simulink model "safety"  (R2014a)
settings: Solver=FixedStepDiscrete  StartTime=0.0  StopTime=inf  FixedStep=2.5e-4  RelTol=1e-3
libraries: simulink x10, xpcethercatlib x5
settings Model: xpc_rtwmakecfg_data=_xpcethercatlib_  Creator=drl  LastModifiedBy=drl
settings OptimizationCC: BlockReduction=off

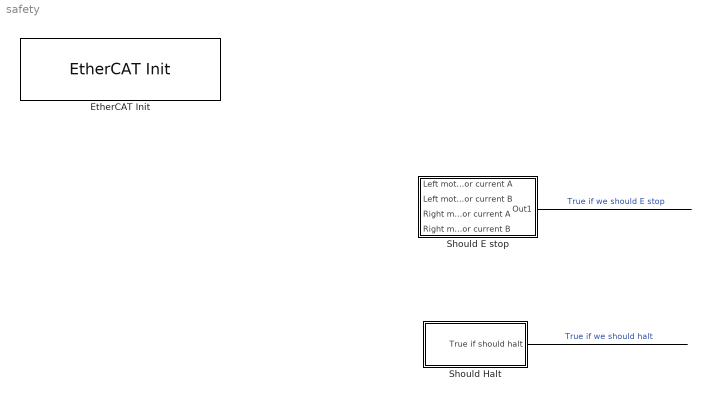
== system safety ==
  "EtherCAT Init " : xpcethercatlib/EtherCAT Init   Priority=0  config_file=C:\Users\drl\Documents\MATLAB\eni_elmo_medulla_4khz.xml  device_id=0  pci_bus=0  pci_slot=0  enaDebug=off  enaDC=on  errLink=off  masterDbg=off  stateChgDbg=off  baseClock=off  masterCfg=off  logFile='c:\dbglog.txt'  sample_time=0.000250
  Should E stop : Subsystem
  Should Halt : Subsystem
  wires:
  Should Halt/1(True if should halt) -> ?  "True if we should halt"
  Should E stop/1(Out1) -> ?  "True if we should E stop"

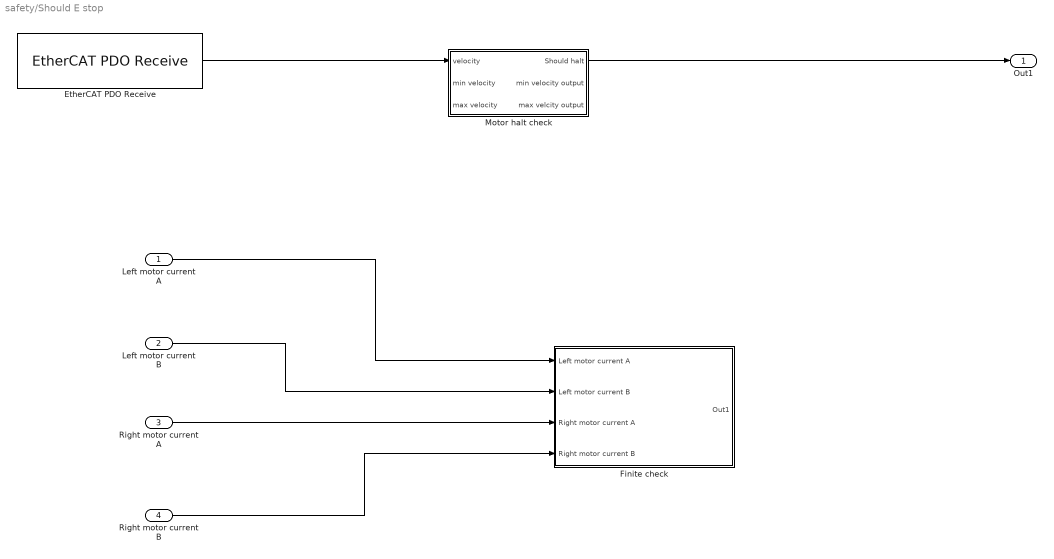
== system safety/Should E stop ==
  Left motor current A : Inport
  Left motor current B : Inport  Port=2
  Right motor current A : Inport  Port=3
  Right motor current B : Inport  Port=4
  EtherCAT PDO Receive : xpcethercatlib/EtherCAT PDO Receive  Priority=2  sig_name=Box 1 (Elmo Drive).Inputs.Position actual value  sig_offset=1064  sig_type=int32  type_size=32  sig_dim=1  device_id=0  sample_time=0.00025
  Finite check : Subsystem
  Motor halt check : Subsystem
  Out1 : Outport
  wires:
  Motor halt check/1(Should halt) -> Out1/1
  EtherCAT PDO Receive/1 -> Motor halt check/1(velocity)
  Left motor current A/1 -> Finite check/1(Left motor current A)
  Left motor current B/1 -> Finite check/2(Left motor current B)
  Right motor current A/1 -> Finite check/3(Right motor current A)
  Right motor current B/1 -> Finite check/4(Right motor current B)

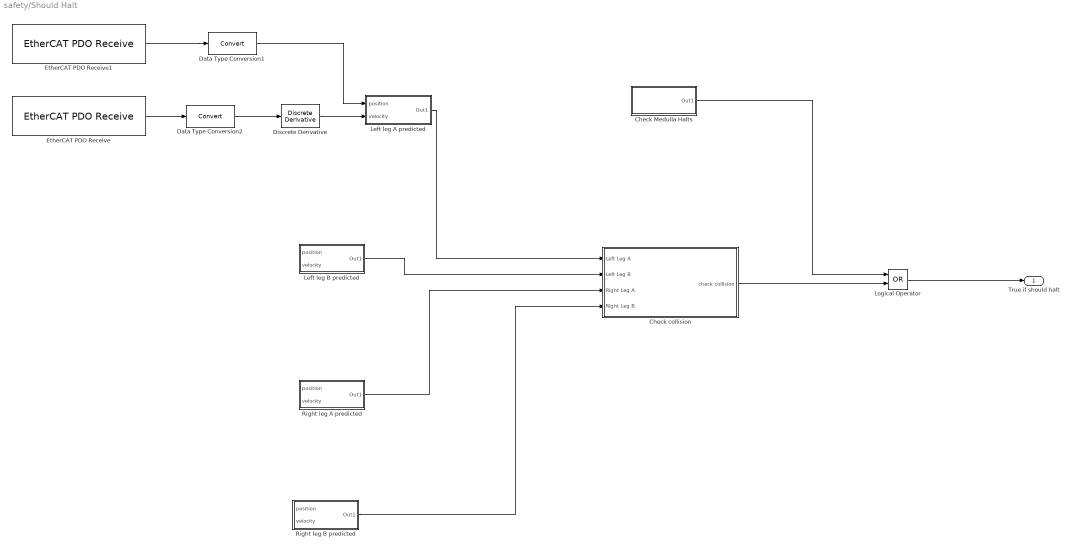
== system safety/Should Halt ==
  Check Medulla Halts : Subsystem
  Check collision : Subsystem
  Data Type Conversion1 : DataTypeConversion
  Data Type Conversion2 : DataTypeConversion
  Discrete Derivative : simulink/Discrete/Discrete Derivative  gainval=1.0  ICPrevScaledInput=0.0  InputProcessing=Inherited  OutMin=[]  OutMax=[]  OutDataType=fixdt(1, 16)  OutScaling=2^-10  DoSatur=off
  EtherCAT PDO Receive : xpcethercatlib/EtherCAT PDO Receive  Priority=2  sig_name=Box 1 (Elmo Drive).Inputs.Position actual value  sig_offset=1064  sig_type=int32  type_size=32  sig_dim=1  device_id=0  sample_time=0.00025
  EtherCAT PDO Receive1 : xpcethercatlib/EtherCAT PDO Receive  Priority=2  sig_name=Drive 1 (Elmo Drive).Inputs.Position actual value  sig_offset=1064  sig_type=int32  type_size=32  sig_dim=1  device_id=0  sample_time=0.00025
  Left leg A predicted : Subsystem
  Left leg B predicted : Subsystem
  Logical Operator : Logic  Operator=OR  AllPortsSameDT=off  OutDataTypeStr=boolean
  Right leg A predicted : Subsystem
  Right leg B predicted : Subsystem
  True if should halt : Outport
  wires:
  Left leg A predicted/1(Out1) -> Check collision/1(Left Leg A)
  Left leg B predicted/1(Out1) -> Check collision/2(Left Leg B)
  Right leg A predicted/1(Out1) -> Check collision/3(Right Leg A)
  Right leg B predicted/1(Out1) -> Check collision/4(Right Leg B)
  Check collision/1(check collision) -> Logical Operator/2
  Check Medulla Halts/1(Out1) -> Logical Operator/1
  Logical Operator/1 -> True if should halt/1
  EtherCAT PDO Receive/1 -> Data Type Conversion2/1
  Data Type Conversion2/1 -> Discrete Derivative/1
  Discrete Derivative/1 -> Left leg A predicted/2(velocity)
  EtherCAT PDO Receive1/1 -> Data Type Conversion1/1
  Data Type Conversion1/1 -> Left leg A predicted/1(position)

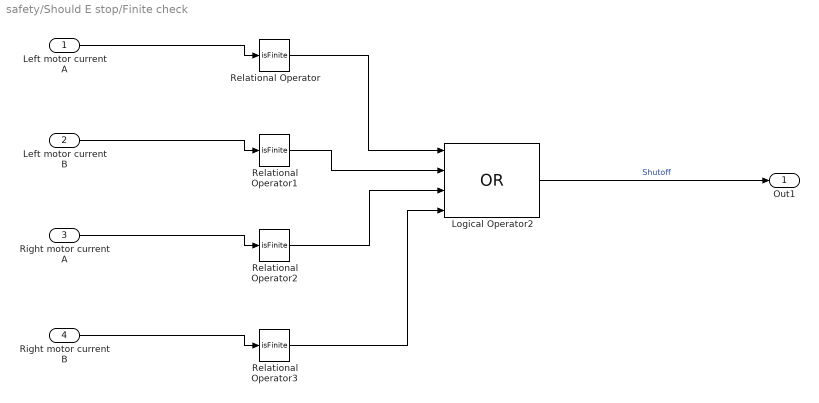
== system safety/Should E stop/Finite check ==
  Left motor current A : Inport
  Left motor current B : Inport  Port=2
  Right motor current A : Inport  Port=3
  Right motor current B : Inport  Port=4
  Logical Operator2 : Logic  Operator=OR  Inputs=4  AllPortsSameDT=off  OutDataTypeStr=boolean
  Relational Operator{,1..3} (4 alike) : RelationalOperator  Operator=isFinite  OutDataTypeStr=boolean
  Out1 : Outport
  wires:
  Logical Operator2/1 -> Out1/1  "Shutoff"
  Left motor current A/1 -> Relational Operator/1
  Left motor current B/1 -> Relational Operator1/1
  Right motor current A/1 -> Relational Operator2/1
  Right motor current B/1 -> Relational Operator3/1
  Relational Operator/1 -> Logical Operator2/1
  Relational Operator1/1 -> Logical Operator2/2
  Relational Operator2/1 -> Logical Operator2/3
  Relational Operator3/1 -> Logical Operator2/4

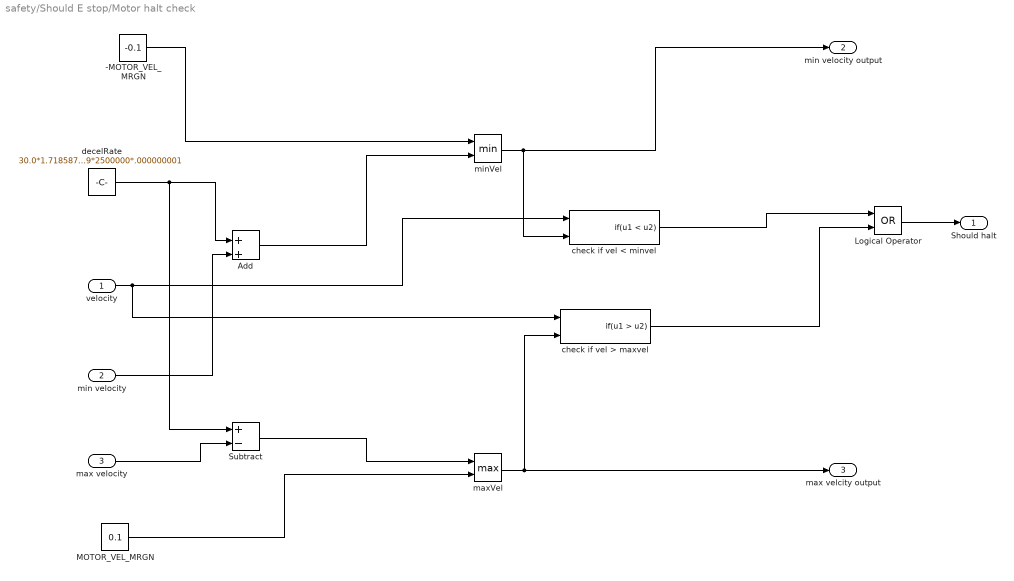
== system safety/Should E stop/Motor halt check ==
  velocity : Inport
  min velocity : Inport  Port=2
  max velocity : Inport  Port=3
  -MOTOR_VEL_MRGN : Constant  Value=-0.1
  Add : Sum  Inputs=+|+
  Logical Operator : Logic  Operator=OR  AllPortsSameDT=off  OutDataTypeStr=boolean
  MOTOR_VEL_MRGN : Constant  Value=0.1
  Subtract : Sum  Inputs=+-
  check if vel < minvel : If  NumInputs=2  IfExpression=u1 < u2  ShowElse=off
  check if vel > maxvel : If  NumInputs=2  IfExpression=u1 > u2  ShowElse=off
  decelRate : Constant  Value=30.0*1.7185879*2500000*.000000001
  maxVel : MinMax  Function=max  Inputs=2
  minVel : MinMax  Inputs=2
  Should halt : Outport
  min velocity output : Outport  Port=2
  max velcity output : Outport  Port=3
  wires:
  -MOTOR_VEL_MRGN/1 -> minVel/1
  min velocity/1 -> Add/2
  decelRate/1 -> Subtract/1, Add/1
  Add/1 -> minVel/2
  max velocity/1 -> Subtract/2
  MOTOR_VEL_MRGN/1 -> maxVel/2
  Subtract/1 -> maxVel/1
  maxVel/1 -> check if vel > maxvel/2, max velcity output/1
  check if vel < minvel/1 -> Logical Operator/1
  minVel/1 -> check if vel < minvel/2, min velocity output/1
  velocity/1 -> check if vel < minvel/1, check if vel > maxvel/1
  check if vel > maxvel/1 -> Logical Operator/2
  Logical Operator/1 -> Should halt/1

== system safety/Should Halt/Check Medulla Halts ==
  Compare To Constant : simulink/Logic and Bit Operations/Compare To Constant  relop===  const=4  OutDataTypeStr=boolean
  EtherCAT PDO Receive : xpcethercatlib/EtherCAT PDO Receive  Priority=2  sig_name=Box 2 (ATRIAS 2.1 Leg (Medulla 1.5)).uController Status.State  sig_offset=600  sig_type=uint8  type_size=8  sig_dim=1  device_id=0  sample_time=0.00025
  Out1 : Outport
  wires:
  EtherCAT PDO Receive/1 -> Compare To Constant/1
  Compare To Constant/1 -> Out1/1

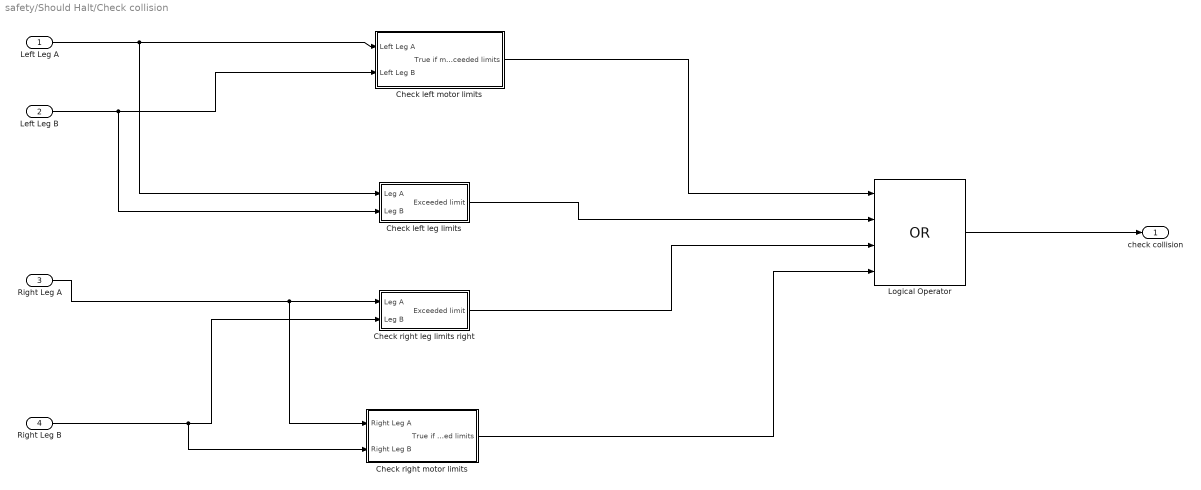
== system safety/Should Halt/Check collision ==
  Left Leg A : Inport
  Left Leg B : Inport  Port=2
  Right Leg A : Inport  Port=3
  Right Leg B : Inport  Port=4
  Check left leg limits : Subsystem
  Check left motor limits : Subsystem
  Check right leg limits right : Subsystem
  Check right motor limits : Subsystem
  Logical Operator : Logic  Operator=OR  Inputs=4  AllPortsSameDT=off  OutDataTypeStr=boolean
  check collision : Outport
  wires:
  Left Leg A/1 -> Check left leg limits/1(Leg A), Check left motor limits/1(Left Leg A)
  Left Leg B/1 -> Check left leg limits/2(Leg B), Check left motor limits/2(Left Leg B)
  Right Leg A/1 -> Check right motor limits/1(Right Leg A), Check right leg limits right/1(Leg A)
  Right Leg B/1 -> Check right motor limits/2(Right Leg B), Check right leg limits right/2(Leg B)
  Check left motor limits/1(True if motor exceeded limits) -> Logical Operator/1
  Check left leg limits/1(Exceeded limit) -> Logical Operator/2
  Check right leg limits right/1(Exceeded limit) -> Logical Operator/3
  Check right motor limits/1(True if motor exceeded limits) -> Logical Operator/4
  Logical Operator/1 -> check collision/1

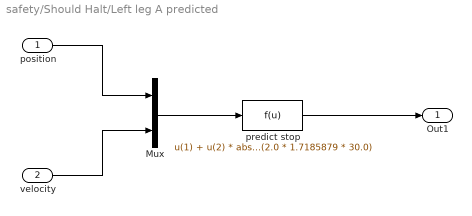
== system safety/Should Halt/Left leg A predicted ==
  position : Inport
  velocity : Inport  Port=2
  Mux : Mux  Inputs=2
  predict stop : Fcn  Expr=u(1) + u(2) * abs(u(2)) / (2.0 * 1.7185879 * 30.0)
  Out1 : Outport
  wires:
  position/1 -> Mux/1
  velocity/1 -> Mux/2
  Mux/1 -> predict stop/1
  predict stop/1 -> Out1/1

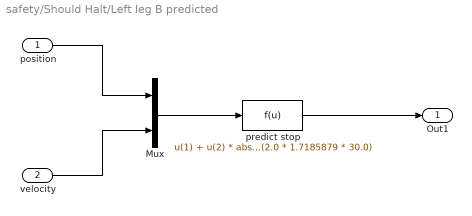
== system safety/Should Halt/Left leg B predicted ==
  position : Inport
  velocity : Inport  Port=2
  Mux : Mux  Inputs=2
  predict stop : Fcn  Expr=u(1) + u(2) * abs(u(2)) / (2.0 * 1.7185879 * 30.0)
  Out1 : Outport
  wires:
  position/1 -> Mux/1
  velocity/1 -> Mux/2
  Mux/1 -> predict stop/1
  predict stop/1 -> Out1/1

== system safety/Should Halt/Right leg A predicted ==
  position : Inport
  velocity : Inport  Port=2
  Mux : Mux  Inputs=2
  predict stop : Fcn  Expr=u(1) + u(2) * abs(u(2)) / (2.0 * 1.7185879 * 30.0)
  Out1 : Outport
  wires:
  position/1 -> Mux/1
  velocity/1 -> Mux/2
  Mux/1 -> predict stop/1
  predict stop/1 -> Out1/1

== system safety/Should Halt/Right leg B predicted ==
  position : Inport
  velocity : Inport  Port=2
  Mux : Mux  Inputs=2
  predict stop : Fcn  Expr=u(1) + u(2) * abs(u(2)) / (2.0 * 1.7185879 * 30.0)
  Out1 : Outport
  wires:
  position/1 -> Mux/1
  velocity/1 -> Mux/2
  Mux/1 -> predict stop/1
  predict stop/1 -> Out1/1

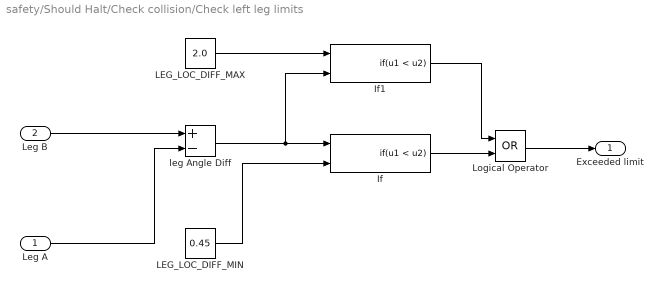
== system safety/Should Halt/Check collision/Check left leg limits ==
  Leg A : Inport
  Leg B : Inport  Port=2
  If : If  NumInputs=2  IfExpression=u1 < u2  ShowElse=off
  If1 : If  NumInputs=2  IfExpression=u1 < u2  ShowElse=off
  LEG_LOC_DIFF_MAX : Constant  Value=2.0
  LEG_LOC_DIFF_MIN : Constant  Value=0.45
  Logical Operator : Logic  Operator=OR  AllPortsSameDT=off  OutDataTypeStr=boolean
  leg Angle Diff : Sum  Inputs=+-
  Exceeded limit : Outport
  wires:
  Leg B/1 -> leg Angle Diff/1
  Leg A/1 -> leg Angle Diff/2
  leg Angle Diff/1 -> If1/2, If/1
  LEG_LOC_DIFF_MIN/1 -> If/2
  If/1 -> Logical Operator/2
  LEG_LOC_DIFF_MAX/1 -> If1/1
  If1/1 -> Logical Operator/1
  Logical Operator/1 -> Exceeded limit/1

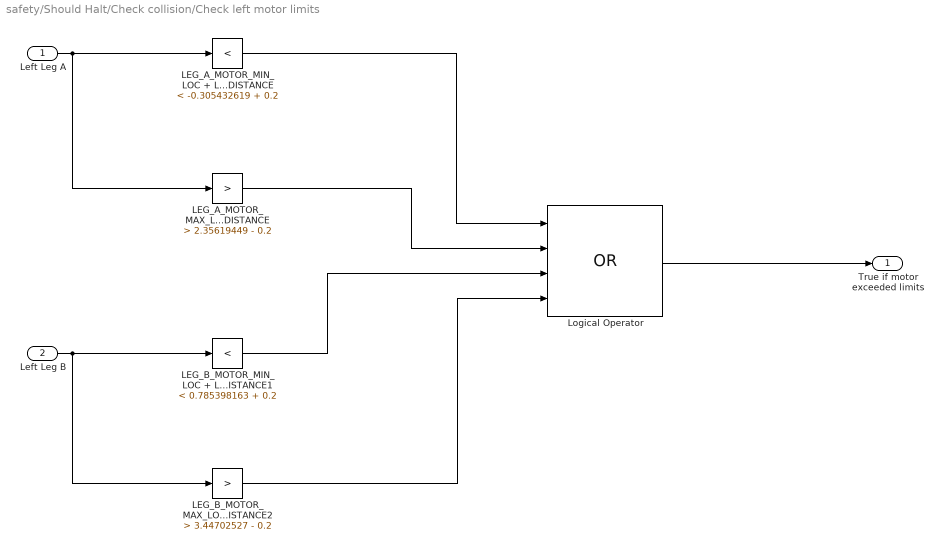
== system safety/Should Halt/Check collision/Check left motor limits ==
  Left Leg A : Inport
  Left Leg B : Inport  Port=2
  LEG_A_MOTOR_MAX_LOC - LEG_LOC_SAFETY_DISTANCE : simulink/Logic and Bit Operations/Compare To Constant  relop=>  const=2.35619449 - 0.2  OutDataTypeStr=boolean
  LEG_A_MOTOR_MIN_LOC + LEG_LOC_SAFETY_DISTANCE : simulink/Logic and Bit Operations/Compare To Constant  relop=<  const=-0.305432619 + 0.2  OutDataTypeStr=boolean
  LEG_B_MOTOR_MAX_LOC - LEG_LOC_SAFETY_DISTANCE2 : simulink/Logic and Bit Operations/Compare To Constant  relop=>  const=3.44702527 - 0.2  OutDataTypeStr=boolean
  LEG_B_MOTOR_MIN_LOC + LEG_LOC_SAFETY_DISTANCE1 : simulink/Logic and Bit Operations/Compare To Constant  relop=<  const=0.785398163 + 0.2  OutDataTypeStr=boolean
  Logical Operator : Logic  Operator=OR  Inputs=4  AllPortsSameDT=off  OutDataTypeStr=boolean
  True if motor exceeded limits : Outport
  wires:
  Left Leg A/1 -> LEG_A_MOTOR_MAX_LOC - LEG_LOC_SAFETY_DISTANCE/1, LEG_A_MOTOR_MIN_LOC + LEG_LOC_SAFETY_DISTANCE/1
  Left Leg B/1 -> LEG_B_MOTOR_MAX_LOC - LEG_LOC_SAFETY_DISTANCE2/1, LEG_B_MOTOR_MIN_LOC + LEG_LOC_SAFETY_DISTANCE1/1
  LEG_A_MOTOR_MIN_LOC + LEG_LOC_SAFETY_DISTANCE/1 -> Logical Operator/1
  LEG_A_MOTOR_MAX_LOC - LEG_LOC_SAFETY_DISTANCE/1 -> Logical Operator/2
  LEG_B_MOTOR_MIN_LOC + LEG_LOC_SAFETY_DISTANCE1/1 -> Logical Operator/3
  LEG_B_MOTOR_MAX_LOC - LEG_LOC_SAFETY_DISTANCE2/1 -> Logical Operator/4
  Logical Operator/1 -> True if motor exceeded limits/1

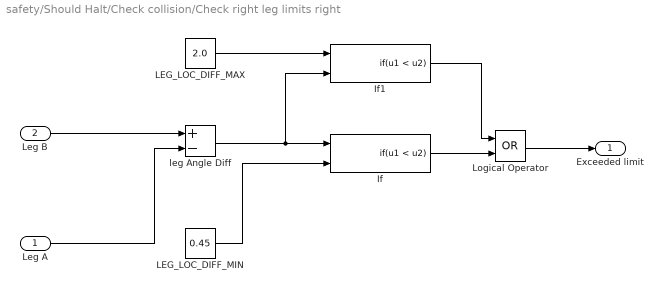
== system safety/Should Halt/Check collision/Check right leg limits right ==
  Leg A : Inport
  Leg B : Inport  Port=2
  If : If  NumInputs=2  IfExpression=u1 < u2  ShowElse=off
  If1 : If  NumInputs=2  IfExpression=u1 < u2  ShowElse=off
  LEG_LOC_DIFF_MAX : Constant  Value=2.0
  LEG_LOC_DIFF_MIN : Constant  Value=0.45
  Logical Operator : Logic  Operator=OR  AllPortsSameDT=off  OutDataTypeStr=boolean
  leg Angle Diff : Sum  Inputs=+-
  Exceeded limit : Outport
  wires:
  Leg B/1 -> leg Angle Diff/1
  Leg A/1 -> leg Angle Diff/2
  leg Angle Diff/1 -> If1/2, If/1
  LEG_LOC_DIFF_MIN/1 -> If/2
  If/1 -> Logical Operator/2
  LEG_LOC_DIFF_MAX/1 -> If1/1
  If1/1 -> Logical Operator/1
  Logical Operator/1 -> Exceeded limit/1

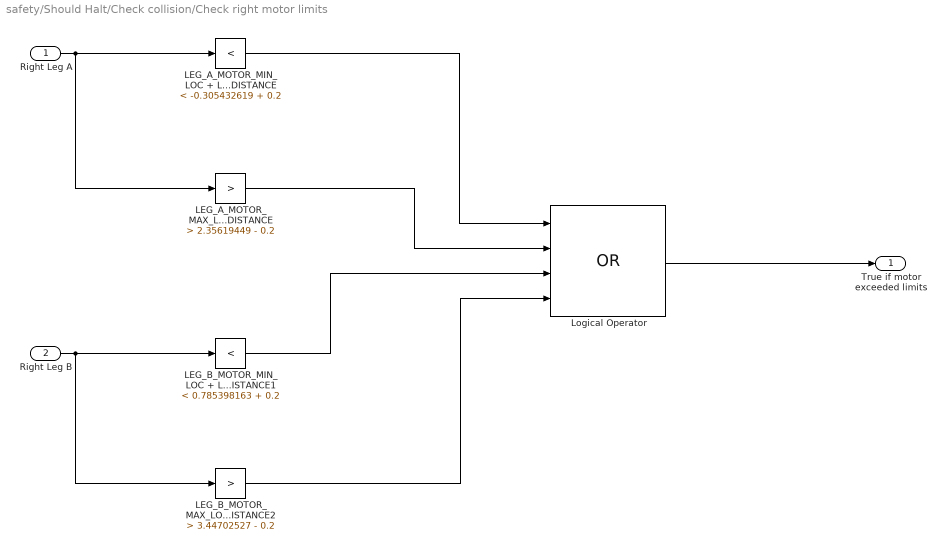
== system safety/Should Halt/Check collision/Check right motor limits ==
  Right Leg A : Inport
  Right Leg B : Inport  Port=2
  LEG_A_MOTOR_MAX_LOC - LEG_LOC_SAFETY_DISTANCE : simulink/Logic and Bit Operations/Compare To Constant  relop=>  const=2.35619449 - 0.2  OutDataTypeStr=boolean
  LEG_A_MOTOR_MIN_LOC + LEG_LOC_SAFETY_DISTANCE : simulink/Logic and Bit Operations/Compare To Constant  relop=<  const=-0.305432619 + 0.2  OutDataTypeStr=boolean
  LEG_B_MOTOR_MAX_LOC - LEG_LOC_SAFETY_DISTANCE2 : simulink/Logic and Bit Operations/Compare To Constant  relop=>  const=3.44702527 - 0.2  OutDataTypeStr=boolean
  LEG_B_MOTOR_MIN_LOC + LEG_LOC_SAFETY_DISTANCE1 : simulink/Logic and Bit Operations/Compare To Constant  relop=<  const=0.785398163 + 0.2  OutDataTypeStr=boolean
  Logical Operator : Logic  Operator=OR  Inputs=4  AllPortsSameDT=off  OutDataTypeStr=boolean
  True if motor exceeded limits : Outport
  wires:
  Right Leg A/1 -> LEG_A_MOTOR_MAX_LOC - LEG_LOC_SAFETY_DISTANCE/1, LEG_A_MOTOR_MIN_LOC + LEG_LOC_SAFETY_DISTANCE/1
  Right Leg B/1 -> LEG_B_MOTOR_MAX_LOC - LEG_LOC_SAFETY_DISTANCE2/1, LEG_B_MOTOR_MIN_LOC + LEG_LOC_SAFETY_DISTANCE1/1
  LEG_A_MOTOR_MIN_LOC + LEG_LOC_SAFETY_DISTANCE/1 -> Logical Operator/1
  LEG_A_MOTOR_MAX_LOC - LEG_LOC_SAFETY_DISTANCE/1 -> Logical Operator/2
  LEG_B_MOTOR_MIN_LOC + LEG_LOC_SAFETY_DISTANCE1/1 -> Logical Operator/3
  LEG_B_MOTOR_MAX_LOC - LEG_LOC_SAFETY_DISTANCE2/1 -> Logical Operator/4
  Logical Operator/1 -> True if motor exceeded limits/1
